simulink model "untitled"  (R2013b)
settings: Solver=ode45  StartTime=0.0  StopTime=10.0  RelTol=1e-3
values from neighbouring files (symbols this model uses):
  x = [x1 ; x]    [inv_pen_digital_controller.m]    (also in test.m = zeros(size(x0, 1), size(time, 2)); worstControl.m = zeros(size(time, 2), size(x0, 1)))
settings Model: Creator=root  LastModifiedBy=Ye
settings DebuggingCC: StateNameClashWarn=warning

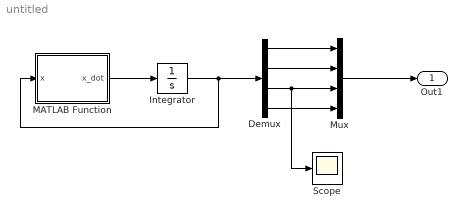
== system untitled ==
  Demux : Demux
  Integrator : Integrator  InitialCondition=x
  MATLAB Function : MATLAB Function  TreatAsAtomicUnit=on
  Mux : Mux
  Scope : Scope
  Out1 : Outport
  wires:
  MATLAB Function/1(x_dot) -> Integrator/1
  Integrator/1 -> MATLAB Function/1(x), Demux/1
  Demux/1 -> Mux/1
  Demux/2 -> Mux/2
  Demux/4 -> Mux/4
  Demux/3 -> Scope/1, Mux/3
  Mux/1 -> Out1/1

== matlab function untitled/MATLAB Function ==
  data: x input; x_dot output
function x_dot = fcn(x)


A = load('A.csv');
B = load('B.csv');
C = load('C.csv');
D = load('D.csv');

x_dot = A*x;
